simulink model "car_model"  (R2022b)
settings: Solver=VariableStepAuto  StartTime=0.0  StopTime=30  RelTol=1e-3
values from neighbouring files (symbols this model uses):
  X = Chassis_Signals.InertFrm.Cg.Disp.X.Data(:)    [Simulation_Data_Parse.m]    (also in Vehicle_Sim_Parse.m)
  Y = Chassis_Signals.InertFrm.Cg.Disp.Y.Data(:)    [Simulation_Data_Parse.m]    (also in Vehicle_Sim_Parse.m)
undefined symbols (not defined in the file or in its folder): ABS_MAX_TORQUE, ABS_MAX_TRQ_CMD, ABS_MIN_TORQUE, acc_IC, ACCELERATION_MAX, ActSuspDutyCycle, Aeq_left, Aeq_right, alpha_error, ang_acc_hystersesis, ang_IC, ang_vel_IC, area_air, axb, battery_current_IC, BATTERY_CURRENT_MAX, BATTERY_CURRENT_MIN, battery_FT_IC, battery_T_IC, BATTERY_TEMPERATURE_MAX, BATTERY_TEMPERATURE_MIN, battery_voltage_IC, BATTERY_VOLTAGE_MAX, BATTERY_VOLTAGE_MIN, Brake_Pressure_IC, ccl_IC, CENTER_STEER_ANGLE_MAX, covA, covarience_matrix_IC, covG, covM, covP, covV, cy_sweep, dB, dcl_IC, DCL_MAX, DCL_MIN, deadband_angle, dIndex, DiscIntNeverNeededParam, disk_abore, driver_t, dt_OFF, dt_ON, dTx, dx, dZ, F0z, forward_look_straight, forward_look_turn, fusion_t, fusion_t_sim, Fz_IC, Fz_sweep, g, gearbox_efficiency, gps_counter_IC, gps_ratio, gr ... (+105)
libraries: fl_lib x62, nesl_utility x16, vehdynlibtire x10, vehdynlibsuspension x8, simulink x5, autolibutils x5, sharedtransform x5, EngineCoolingComponents_lib x4, slpidlib x3, SimscapeFluids_lib x3, dspstat3 x2, shared6dof x2
(part 2 of 10)

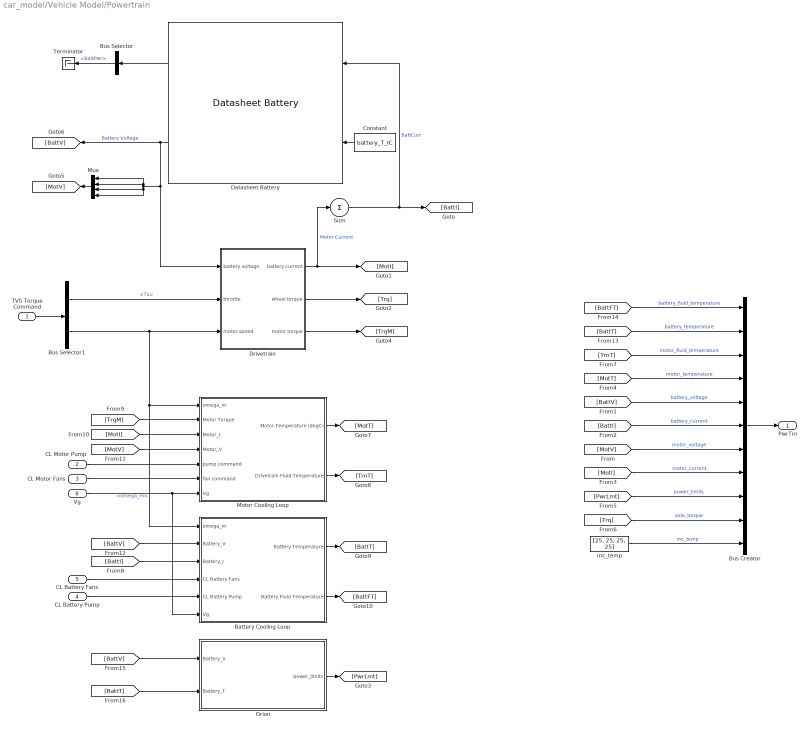
== system car_model/Vehicle Model/Powertrain ==
  TVS Torque Command : Inport
  CL Motor Pump : Inport  Port=2
  CL Motor Fans : Inport  Port=3
  CL Battery Pump : Inport  Port=4
  CL Battery Fans : Inport  Port=5
  Vg : Inport  Port=6
  Battery Cooling Loop : Subsystem
  Bus Creator : BusCreator  Inputs=11
  Bus Selector : BusSelector  OutputSignals=BattPwr
  Bus Selector1 : BusSelector  OutputSignals=Tx,omega_m
  Constant : Constant  Value=battery_T_IC
  Datasheet Battery : autolibdatasheetbattery/Datasheet Battery  CapacityCtrl=Parameter  OutputVlt=Filtered  BattChargeMax=BattCap  Em=Em  CapLUTBp=SOC  RInt=RESISTANCE  BattTempBp=TEMPERATURE  CapSOCBp=SOC  Ns=Ns  Np=Np  BattCapInit=BattCap_I  Tc=Battery_tau  Vinit=battery_voltage_IC  RefBlkName='autolibdatasheetbattery/Datasheet Battery'
  Drivetrain : Subsystem
  Motor Cooling Loop : Subsystem
  Mux : Mux
  Orion : Subsystem
  Sum : Sum  Inputs=+
  Terminator : Terminator
  mc_temp : Constant  Value=[25, 25, 25, 25]
  PwrTrn : Outport
  wires:
  [BattT] -> Orion/2(Battery_T)
  [Trq] -> Bus Creator/10  "axle_torque"
  [TrnT] -> Bus Creator/3  "motor_fluid_temperature"
  Vg/1 -> Motor Cooling Loop/7(Vg), Battery Cooling Loop/6(Vg)
  CL Battery Fans/1 -> Battery Cooling Loop/4(CL Battery Fans)
  [MotT] -> Bus Creator/4  "motor_temperature"
  Battery Cooling Loop/2(Battery Fluid Temperature) -> [BattFT]
  [BattI] -> Bus Creator/6  "battery_current"
  [MotI] -> Bus Creator/8  "motor_current"
  [MotV] -> Motor Cooling Loop/4(Motor_V)
  Motor Cooling Loop/2(Drivetrain Fluid Temperature) -> [TrnT]
  Mux/1 -> [MotV]
  CL Battery Pump/1 -> Battery Cooling Loop/5(CL Battery Pump)
  Bus Selector1/2 -> Drivetrain/3(motor speed), Motor Cooling Loop/1(omega_m), Battery Cooling Loop/1(omega_m)  "<omega_m>"
  Bus Selector1/1 -> Drivetrain/2(throttle)  "<Tx>"
  CL Motor Pump/1 -> Motor Cooling Loop/5(pump command)
  Battery Cooling Loop/1(Battery Temperature) -> [BattT]
  Sum/1 -> [BattI], Datasheet Battery/1  "BattCurr"
  Datasheet Battery/1 -> Bus Selector/1
  [BattI] -> Battery Cooling Loop/3(Battery_I)
  [BattV] -> Orion/1(Battery_V)
  Bus Selector/1 -> Terminator/1  "<BattPwr>"
  Motor Cooling Loop/1(Motor Temperature (degC)) -> [MotT]
  Datasheet Battery/2 -> Drivetrain/1(battery voltage), Mux/3, Mux/4, Mux/2, Mux/1, [BattV]  "Battery Voltage"
  [MotV] -> Bus Creator/7  "motor_voltage"
  [BattV] -> Bus Creator/5  "battery_voltage"
  [MotI] -> Motor Cooling Loop/3(Motor_I)
  [BattV] -> Battery Cooling Loop/2(Battery_V)
  [BattFT] -> Bus Creator/1  "battery_fluid_temperature"
  Drivetrain/1(battery current) -> [MotI], Sum/1  "Motor Current"
  Constant/1 -> Datasheet Battery/2
  Bus Creator/1 -> PwrTrn/1
  CL Motor Fans/1 -> Motor Cooling Loop/6(fan command)
  [PwrLmt] -> Bus Creator/9  "power_limits"
  [BattT] -> Bus Creator/2  "battery_temperature"
  Orion/1(power_limits) -> [PwrLmt]
  [TrqM] -> Motor Cooling Loop/2(Motor Torque)
  mc_temp/1 -> Bus Creator/11  "mc_temp"
  TVS Torque Command/1 -> Bus Selector1/1
  Drivetrain/2(wheel torque) -> [Trq]
  Drivetrain/3(motor torque) -> [TrqM]

== system car_model/Vehicle Model/Suspension ==
  Steering : Inport
  Wheel : Inport  Port=2
  Vehicle : Inport  Port=3
  Double Wishbone Suspension : Subsystem  VariantControl=1
      mask Display: image('suspdw.png');
  Independent Mapped Front Suspension Mapped Solid Axle Rear Suspension : Subsystem  VariantControl=2
      mask Display: image([imread('suspindmap.png');imread('suspsamap.png')]);
  Kinematics and Compliance Independent Suspension : Subsystem  VariantControl=6
      mask Display: image('suspkandc.png');
  MacPherson Front Suspension Solid Axle Rear Suspension : Subsystem  VariantControl=3
      mask Display: image([imread('suspmacp.png');imread('suspsacoil.png')]);
  MacPherson Suspension : Subsystem  VariantControl=4
      mask Display: image('suspmacp.png');
  Mapped Suspension : Subsystem  VariantControl=5
      mask Display: image('suspindmap.png');
  Suspension : Outport  VectorParamsAs1DForOutWhenUnconnected=off
  Suspension1 : Outport  Port=2  VectorParamsAs1DForOutWhenUnconnected=off
  Veh : Outport  Port=3  VectorParamsAs1DForOutWhenUnconnected=off

== system car_model/Vehicle Model/Vehicle ==
  Suspension : Inport
  6DOF : Subsystem  VariantControl=1
  Constant : Constant  Value=[0 0 0]
  VehFdbk : Outport  VectorParamsAs1DForOutWhenUnconnected=off
  wires:
  6DOF/1(VehFdbk) -> VehFdbk/1  "VehFdbk"
  Constant/1 -> 6DOF/2(Wind)
  Suspension/1 -> 6DOF/1(Suspension)

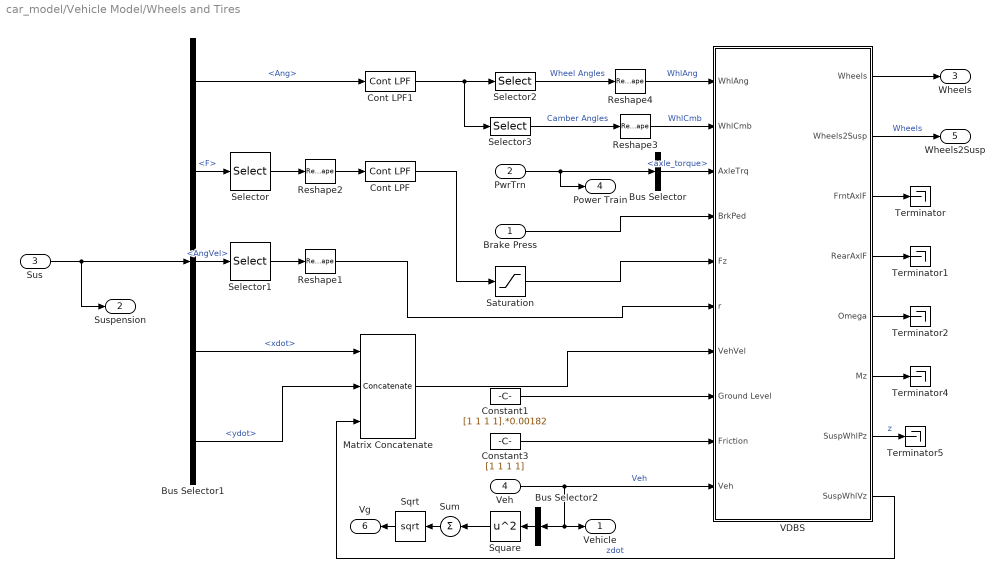
== system car_model/Vehicle Model/Wheels and Tires ==
  Brake Press : Inport  Unit=Pa
  PwrTrn : Inport  Port=2
  Sus : Inport  Port=3
  Veh : Inport  Port=4
  Bus Selector : BusSelector  OutputSignals=axle_torque
  Bus Selector1 : BusSelector  OutputSignals=Whl.Ang,Whl.F,Whl.AngVel,Whl.xdot,Whl.ydot
  Bus Selector2 : BusSelector  OutputSignals=BdyFrm.Cg.Vel.xdot,BdyFrm.Cg.Vel.ydot  OutputAsBus=on
  Constant1 : Constant  Value=[1 1 1 1].*0.00182
  Constant3 : Constant  Value=[1 1 1 1]
  Cont LPF : autolibutils/Cont LPF  wc=100*2*pi  AbsoluteTolerance=auto  aMode=2
  Cont LPF1 : autolibutils/Cont LPF  wc=100*2*pi  AbsoluteTolerance=auto  aMode=2
  Matrix Concatenate : Concatenate  NumInputs=3  Mode=Multidimensional array
  Reshape{1..4} (4 alike) : Reshape
  Saturation : Saturate  UpperLimit=inf  LowerLimit=-10*9.81*2000  ZeroCross=off
  Selector : Selector  NumberOfDimensions=2  InputPortWidth=3  IndexOptions=Index vector (dialog),Select all  Indices=[3],1  OutputSizes=1,1
  Selector1 : Selector  NumberOfDimensions=2  InputPortWidth=1  IndexOptions=Index vector (dialog),Select all  Indices=[3],1  OutputSizes=1,1
  Selector2 : Selector  NumberOfDimensions=2  InputPortWidth=3  IndexOptions=Index vector (dialog),Select all  Indices=3,1  OutputSizes=1,1
  Selector3 : Selector  NumberOfDimensions=2  InputPortWidth=3  IndexOptions=Index vector (dialog),Select all  Indices=1,1  OutputSizes=1,1
  Sqrt : Sqrt
  Square : Math  Operator=square
  Sum : Sum  Inputs=+
  Terminator{,1..2,4..5} (5 alike) : Terminator
  VDBS : Subsystem  VariantControl=0
  Vehicle : Outport  VectorParamsAs1DForOutWhenUnconnected=off
  Suspension : Outport  Port=2  VectorParamsAs1DForOutWhenUnconnected=off
  Wheels : Outport  Port=3  VectorParamsAs1DForOutWhenUnconnected=off
  Power Train : Outport  Port=4  VectorParamsAs1DForOutWhenUnconnected=off
  Wheels2Susp : Outport  Port=5  VectorParamsAs1DForOutWhenUnconnected=off
  Vg : Outport  Port=6  VectorParamsAs1DForOutWhenUnconnected=off
  wires:
  Bus Selector1/2 -> Selector/1  "<F>"
  VDBS/3(FrntAxlF) -> Terminator/1
  VDBS/4(RearAxlF) -> Terminator1/1
  VDBS/6(Mz) -> Terminator4/1
  Selector1/1 -> Reshape1/1
  Matrix Concatenate/1 -> VDBS/7(VehVel)
  PwrTrn/1 -> Power Train/1, Bus Selector/1
  Reshape4/1 -> VDBS/1(WhlAng)  "WhlAng"
  Reshape3/1 -> VDBS/2(WhlCmb)  "WhlCmb"
  Selector/1 -> Reshape2/1
  Saturation/1 -> VDBS/5(Fz)
  Constant1/1 -> VDBS/8(Ground Level)
  VDBS/8(SuspWhlVz) -> Matrix Concatenate/3  "zdot"
  Bus Selector1/1 -> Cont LPF1/1  "<Ang>"
  Selector3/1 -> Reshape3/1  "Camber Angles"
  Sus/1 -> Suspension/1, Bus Selector1/1
  Bus Selector1/4 -> Matrix Concatenate/1  "<xdot>"
  Bus Selector1/5 -> Matrix Concatenate/2  "<ydot>"
  VDBS/7(SuspWhlPz) -> Terminator5/1  "z"
  Reshape2/1 -> Cont LPF/1
  Bus Selector1/3 -> Selector1/1  "<AngVel>"
  Reshape1/1 -> VDBS/6(r)
  Brake Press/1 -> VDBS/4(BrkPed)
  Constant3/1 -> VDBS/9(Friction)
  Cont LPF/1 -> Saturation/1
  Cont LPF1/1 -> Selector3/1, Selector2/1
  Selector2/1 -> Reshape4/1  "Wheel Angles"
  Veh/1 -> Vehicle/1, Bus Selector2/1, VDBS/10(Veh)  "Veh"
  VDBS/2(Wheels2Susp) -> Wheels2Susp/1  "Wheels"
  VDBS/1(Wheels) -> Wheels/1
  Bus Selector/1 -> VDBS/3(AxleTrq)  "<axle_torque>"
  VDBS/5(Omega) -> Terminator2/1
  Bus Selector2/1 -> Square/1
  Square/1 -> Sum/1
  Sum/1 -> Sqrt/1
  Sqrt/1 -> Vg/1

== system car_model/Control Systems/TVS/Current Limiting ==
  max_K : Inport
  omega : Inport  Port=2
  Tx : Inport  Port=3
  Divide : Product  Inputs=/**
  Gain : Gain  Gain=1./ABS_MAX_TORQUE
  Gain1 : Gain  Gain=PER23_gr
  Gain2 : Gain  Gain=MOTOR_ENABLE
  GreaterThan : RelationalOperator  Operator=<  OutDataTypeStr=boolean  RndMeth=Simplest  InputSameDT=off
  Max : MinMax  Function=max
  Max K : Lookup_n-D  NumberOfTableDimensions=1  BreakpointsForDimension1=[0 675]  Table=[0.05 1]  ExtrapMethod=Clip  UseLastTableValue=on  InternalRulePriority=Speed  RndMeth=Simplest
  Min K : Lookup_n-D  NumberOfTableDimensions=1  BreakpointsForDimension1=[0 100 200 1150]  IndexSearchMethod=Linear search  Table=[0 0 0.1 1]  ExtrapMethod=Clip  UseLastTableValue=on  InternalRulePriority=Speed  RndMeth=Simplest
  Product : Product
  Sum : Sum  Inputs=+
  Sum1 : Sum  Inputs=+|+
  Sum2 : Sum  Inputs=|+-
  Switch : Switch  Criteria=u2 > Threshold  SaturateOnIntegerOverflow=off  InputSameDT=off
  K_Actual : Outport
  wires:
  max_K/1 -> Divide/3, GreaterThan/1
  Switch/1 -> K_Actual/1
  Gain/1 -> Product/1
  Tx/1 -> Gain/1
  GreaterThan/1 -> Sum/1
  Sum/1 -> Switch/2
  omega/1 -> Gain1/1
  Min K/1 -> Gain2/1, Sum2/2
  Max K/1 -> Sum2/1
  Sum2/1 -> Product/2
  Product/1 -> Sum1/1
  Sum1/1 -> Switch/3, Divide/2, Max/1, GreaterThan/2
  Max/1 -> Divide/1
  Divide/1 -> Switch/1
  Gain1/1 -> Min K/1, Max K/1
  Gain2/1 -> Sum1/2

== system car_model/Control Systems/TVS/Optimization ==
  note: reduce this limit?
  driver_input : Inport  OutDataTypeStr=double
  obj_gain : Inport  Port=2
  b : Inport  Port=3  OutDataTypeStr=double
  ub : Inport  Port=4  OutDataTypeStr=double
  lb : Inport  Port=5  OutDataTypeStr=double
  Aeq : Inport  Port=6  OutDataTypeStr=double
  beq : Inport  Port=7  OutDataTypeStr=double
  A Dot : DotProduct  OutDataTypeStr=double
  Aeq Dot : DotProduct  OutDataTypeStr=double
  C Caller : CCaller  FunctionName=bigM_func  PortSpecificationStruct="%)30     .    N\"X   8    (     @         %    \"    !P    !     0         %  0 \"0    $    _    07)G3F%M90  4&]R=$YA;64 4V-O<&4     26YD97@     5'EP90      4VEZ90      27-';&]B86P   X    P    !@    @    $          4    (     0    ,    !         !   P!O=70 #@   #     &    \"     0         !0    @    !     P    $         $  # &]U=  .    .     8    (    !          %    \"     $    &     0         0  ...(+15750 chars)"
  Constant : Constant  Value=TVS_ENABLE
  Constant1 : Constant  Value=[1 1 1 1]
  Demux{,1..4} (5 alike) : Demux
  Switch : Switch  Criteria=u2 > Threshold  SaturateOnIntegerOverflow=off  InputSameDT=off
  Tx_RAW_demux : Mux
  Tx_choose : Switch  Criteria=u2 > Threshold  Threshold=2  OutDataTypeStr=double  SaturateOnIntegerOverflow=off  InputSameDT=off
  Tx_deadband : DeadZone  LowerValue=-10*dTx  UpperValue=10*dTx  SaturateOnIntegerOverflow=off
  Tx_equal_gain : Gain  Gain=ABS_MAX_TORQUE.*MOTOR_ENABLE  OutDataTypeStr=double
  Tx_equal_offset : Bias  Bias=ABS_MAX_TORQUE  SaturateOnIntegerOverflow=off
  Tx_initial : Constant  Value=Tx_I  OutDataTypeStr=double
  Tx_reverse_offset : Bias  Bias=-ABS_MAX_TORQUE  SaturateOnIntegerOverflow=off
  b Add : Sum  OutDataTypeStr=double
  beq Add : Sum  OutDataTypeStr=double
  lb_offset : Bias  Bias=ABS_MAX_TORQUE  SaturateOnIntegerOverflow=off
  optimization_offset_A : Constant  Value=ABS_MAX_TORQUE  OutDataTypeStr=double
  optimization_offset_Aeq : Constant  Value=ABS_MAX_TORQUE  OutDataTypeStr=double
  ub_offset : Bias  Bias=ABS_MAX_TORQUE  SaturateOnIntegerOverflow=off
  yaw_error_limit : Constant  Value=yaw_error_limit  OutDataTypeStr=double
  Tx : Outport
  exitflag : Outport  Port=2
  wires:
  C Caller/1 -> Tx_choose/2, exitflag/1  "exitflag"
  lb/1 -> lb_offset/1  "lb"
  ub/1 -> ub_offset/1  "ub"
  C Caller/2 -> Tx_RAW_demux/1  "TFL"
  C Caller/5 -> Tx_RAW_demux/4  "TRR"
  C Caller/4 -> Tx_RAW_demux/3  "TRL"
  C Caller/3 -> Tx_RAW_demux/2  "TFR"
  Demux/1 -> C Caller/1  "obj_FL"
  Demux/2 -> C Caller/2  "obj_FR"
  Demux/3 -> C Caller/3  "obj_RL"
  Demux/4 -> C Caller/4  "obj_RR"
  Tx_initial/1 -> C Caller/23, C Caller/24, C Caller/25, C Caller/26  "Tx_initial"
  Demux1/1 -> C Caller/19  "ub_FL"
  Demux1/2 -> C Caller/20  "ub_FR"
  Demux1/3 -> C Caller/21  "ub_RL"
  Demux1/4 -> C Caller/22  "ub_RR"
  Demux2/1 -> C Caller/15  "lb_FL"
  Demux2/2 -> C Caller/16  "lb_FR"
  Demux2/3 -> C Caller/17  "lb_RL"
  Demux2/4 -> C Caller/18  "lb_RR"
  Demux3/3 -> C Caller/13  "Aeq_RL"
  Demux3/2 -> C Caller/12  "Aeq_FR"
  Demux3/1 -> C Caller/11  "Aeq_FL"
  Demux3/4 -> C Caller/14  "Aeq_RR"
  Demux4/1 -> C Caller/6  "A_FL"
  Demux4/2 -> C Caller/7  "A_FR"
  Demux4/3 -> C Caller/8  "A_RL"
  Demux4/4 -> C Caller/9  "A_RR"
  ub_offset/1 -> Demux1/1  "ub_b"
  optimization_offset_Aeq/1 -> Aeq Dot/1  "offset"
  optimization_offset_A/1 -> A Dot/1  "offset"
  beq/1 -> beq Add/1  "beq"
  Aeq Dot/1 -> beq Add/2  "Aeq_b"
  b/1 -> b Add/1  "b"
  A Dot/1 -> b Add/2
  yaw_error_limit/1 -> C Caller/27  "yaw_error_limit"
  Tx_RAW_demux/1 -> Tx_choose/1  "Tx_RAW_TV"
  Constant1/1 -> Demux4/1, A Dot/2  "A"
  b Add/1 -> C Caller/5  "b_b"
  obj_gain/1 -> Demux/1  "obj_gain"
  lb_offset/1 -> Demux2/1  "lb_b"
  Aeq/1 -> Demux3/1, Aeq Dot/2  "Aeq"
  beq Add/1 -> C Caller/10  "beq_b"
  Tx_deadband/1 -> Tx/1  "Tx"
  Tx_reverse_offset/1 -> Tx_deadband/1
  driver_input/1 -> Tx_equal_gain/1
  Tx_choose/1 -> Switch/1
  Tx_equal_gain/1 -> Tx_equal_offset/1  "Tx_equal"
  Tx_equal_offset/1 -> Switch/3, Tx_choose/3
  Switch/1 -> Tx_reverse_offset/1
  Constant/1 -> Switch/2

== system car_model/Control Systems/TVS/Power Controller ==
  note: Max Throttle as Limit or Max Current as limit?
  note: Tune the endpoints
  vel : Inport  OutDataTypeStr=double
  battery_voltage : Inport  Port=2
  dcl : Inport  Port=3  OutDataTypeStr=double  LockScale=on
  ccl : Inport  Port=4  OutDataTypeStr=double  LockScale=on
  driver_input : Inport  Port=5  OutDataTypeStr=double  LockScale=on
  motor_temp : Inport  Port=6
  mc_temp : Inport  Port=7
  omega : Inport  Port=8
  In9 : Inport  Port=9
  Constant2 : Constant  Value=[0 0 0 0]  OutDataTypeStr=double
  Constant3 : Constant  Value=ABS_MAX_TORQUE
  Current to RAW Throttle : Gain  Gain=1/(2*MOTOR_CURRENT_LIMIT)
  Gain : Gain  Gain=2*MOTOR_CURRENT_LIMIT
  Gain1 : Gain  Gain=ABS_MAX_TRQ_CMD
  Gain4 : Gain  Gain=-MOTOR_ENABLE  ParamDataTypeStr=double  OutDataTypeStr=Inherit: Inherit via back propagation
  Gain8 : Gain  Gain=MOTOR_ENABLE  ParamDataTypeStr=double  OutDataTypeStr=Inherit: Inherit via back propagation
  Max : MinMax  Function=max
  Max Torque : Saturate  UpperLimit=ABS_MAX_TORQUE  LowerLimit=dTx  OutDataTypeStr=Inherit: Inherit via back propagation
  Max1 : MinMax  Function=max
  Min Torque : Saturate  UpperLimit=ABS_MIN_TORQUE  LowerLimit=0  OutDataTypeStr=Inherit: Inherit via back propagation
  Minimum : MinMax  Inputs=4
  Saturation : Saturate  UpperLimit=ABS_MAX_TRQ_CMD  LowerLimit=dTx*10
  Selector : Selector  InputPortWidth=4  IndexOptions=Index vector (dialog)  Indices=4  OutputSizes=1
  Switch1 : Switch  Threshold=min_velocity_regen  OutDataTypeStr=Inherit: Inherit via back propagation  SaturateOnIntegerOverflow=off  InputSameDT=off
  Temperature to Motor Controller Current Limit Map : Lookup_n-D  NumberOfTableDimensions=1  BreakpointsForDimension1=motorControllerCurve(:,1)  IndexSearchMethod=Evenly spaced points  Table=motorControllerCurve(:,2)  ExtrapMethod=Clip  UseLastTableValue=on  InternalRulePriority=Speed  RndMeth=Simplest
  Temperature to Motor Current Limit Map : Lookup_n-D  NumberOfTableDimensions=1  BreakpointsForDimension1=motorTempX  IndexSearchMethod=Evenly spaced points  Table=motorTempCurve  ExtrapMethod=Clip  UseLastTableValue=on  InternalRulePriority=Speed  RndMeth=Simplest
  Terminator : Terminator
  Terminator1 : Terminator
  Terminator2 : Terminator
  b : Outport  OutDataTypeStr=double  LockScale=on
  max_K : Outport  Port=2  OutDataTypeStr=double  LockScale=on
  ub : Outport  Port=3  OutDataTypeStr=double  LockScale=on
  lb : Outport  Port=4  OutDataTypeStr=double  LockScale=on
  wires:
  Max1/1 -> Temperature to Motor Controller Current Limit Map/1
  Temperature to Motor Current Limit Map/1 -> Minimum/2  "Total Motor Current Limit (A)"
  battery_voltage/1 -> Terminator1/1
  Gain8/1 -> Max Torque/1
  Constant3/1 -> Gain4/1, Gain8/1
  Saturation/1 -> b/1  "Limited Total Torque Request (Nm)"
  Max/1 -> Temperature to Motor Current Limit Map/1
  Gain4/1 -> Min Torque/1
  Constant2/1 -> Switch1/3  "Abs Min Torque CMD"
  Selector/1 -> Switch1/2  "Planer Vcog (m/s)"
  motor_temp/1 -> Max/1  "[FL FR RL RR] Motor Temperature (degC)"
  ccl/1 -> Terminator/1
  driver_input/1 -> Gain/1, Gain1/1  "RAW Throttle"
  Max Torque/1 -> ub/1  "Max Individual Motor Torque (Nm)"
  Gain/1 -> Minimum/1
  mc_temp/1 -> Max1/1  "[FL FR RL RR] Motor Controller Temperature (degC)"
  dcl/1 -> Minimum/4  "Discharge Current Limit (A)"
  vel/1 -> Selector/1  "[Vx Vy Vcog]"
  Temperature to Motor Controller Current Limit Map/1 -> Minimum/3  "Total Motor Controller Current Limit (A)"
  Min Torque/1 -> Switch1/1
  Switch1/1 -> lb/1  "Min Individual Motor Torque (Nm)"
  Minimum/1 -> Current to RAW Throttle/1  "Max Allowed Current (A)"
  omega/1 -> Terminator2/1
  Gain1/1 -> Saturation/1
  Current to RAW Throttle/1 -> max_K/1  "Torque CMD (none)"

== system car_model/Control Systems/TVS/Traction Controller ==
  Fz : Inport  OutDataTypeStr=double  LockScale=on
  vel : Inport  Port=2  OutDataTypeStr=double  LockScale=on
  ang_vel : Inport  Port=3  OutDataTypeStr=double  LockScale=on
  CCSA : Inport  Port=4
  omega : Inport  Port=5
  1-D Lookup Table : Lookup_n-D  NumberOfTableDimensions=1  BreakpointsForDimension1=Fz_sweep  Table=cy_sweep  InternalRulePriority=Speed  RndMeth=Simplest
  1-D Lookup Table1 : Lookup_n-D  NumberOfTableDimensions=1  BreakpointsForDimension1=Fz_sweep  Table=my_sweep  InternalRulePriority=Speed  RndMeth=Simplest
  1-D Lookup Table2 : Lookup_n-D  NumberOfTableDimensions=1  BreakpointsForDimension1=Fz_sweep  Table=kx_sweep  InternalRulePriority=Speed  RndMeth=Simplest
  1-D Lookup Table3 : Lookup_n-D  NumberOfTableDimensions=1  BreakpointsForDimension1=Fz_sweep  Table=mx_sweep  InternalRulePriority=Speed  RndMeth=Simplest
  Compute SA : Subsystem
  Compute SL : Subsystem
  Compute SL Fake : Subsystem
  Constant : Constant
  Constant1 : Constant  Value=[1 1 1 1].*low_V_SA
  Constant2 : Constant  Value=TRACTION_ENABLE
  Divide : Product  Inputs=**//
  Divide1 : Product  Inputs=**//
  Gain : Gain  Gain=gr./RE
  Selector : Selector  InputPortWidth=4  IndexOptions=Index vector (dialog)  Indices=4  OutputSizes=1
  Selector1 : Selector  InputPortWidth=4  IndexOptions=Index vector (dialog)  Indices=4  OutputSizes=1
  Sqrt : Sqrt
  Square : Math  Operator=square
  Square1 : Math  Operator=square
  Steering Model : Subsystem
  Sum : Sum  Inputs=|++
  Switch : Switch  Criteria=u2 > Threshold  Threshold=Vth  SaturateOnIntegerOverflow=off  InputSameDT=off
  Switch1 : Switch  Criteria=u2 > Threshold  Threshold=Vth  SaturateOnIntegerOverflow=off  InputSameDT=off
  Switch2 : Switch  Criteria=u2 > Threshold  SaturateOnIntegerOverflow=off  InputSameDT=off
  obj_gain : Outport
  wires:
  Gain/1 -> obj_gain/1  "obj_gain"
  Constant/1 -> Gain/1, Switch2/3
  Sum/1 -> Sqrt/1
  Divide/1 -> Square/1  "a_bar"
  1-D Lookup Table/1 -> Divide/2
  1-D Lookup Table1/1 -> Divide/3
  Fz/1 -> 1-D Lookup Table1/1, Divide/4, 1-D Lookup Table2/1, 1-D Lookup Table3/1, Divide1/4, 1-D Lookup Table/1
  Divide1/1 -> Square1/1  "s_bar"
  1-D Lookup Table2/1 -> Divide1/2
  1-D Lookup Table3/1 -> Divide1/3
  Switch/1 -> Divide1/1
  Switch1/1 -> Divide/1
  Compute SL Fake/1(SL_fake) -> Switch/3
  Compute SL/1(Out1) -> Switch/1
  Compute SA/1(Out1) -> Switch1/1, Compute SL/1(In1)
  vel/1 -> Compute SL/3(Vg), Selector/1, Compute SL Fake/2(Vg), Selector1/1, Compute SA/3(Vg)
  ang_vel/1 -> Compute SA/2(ang_vel)
  omega/1 -> Compute SL Fake/1(omega), Compute SL/2(omega)
  Steering Model/1(steering) -> Compute SA/1(steering)
  Constant1/1 -> Switch1/3
  Sqrt/1 -> Switch2/1
  Constant2/1 -> Switch2/2
  Selector/1 -> Switch/2
  Selector1/1 -> Switch1/2
  Square/1 -> Sum/1
  Square1/1 -> Sum/2
  CCSA/1 -> Steering Model/1(steering_angle)

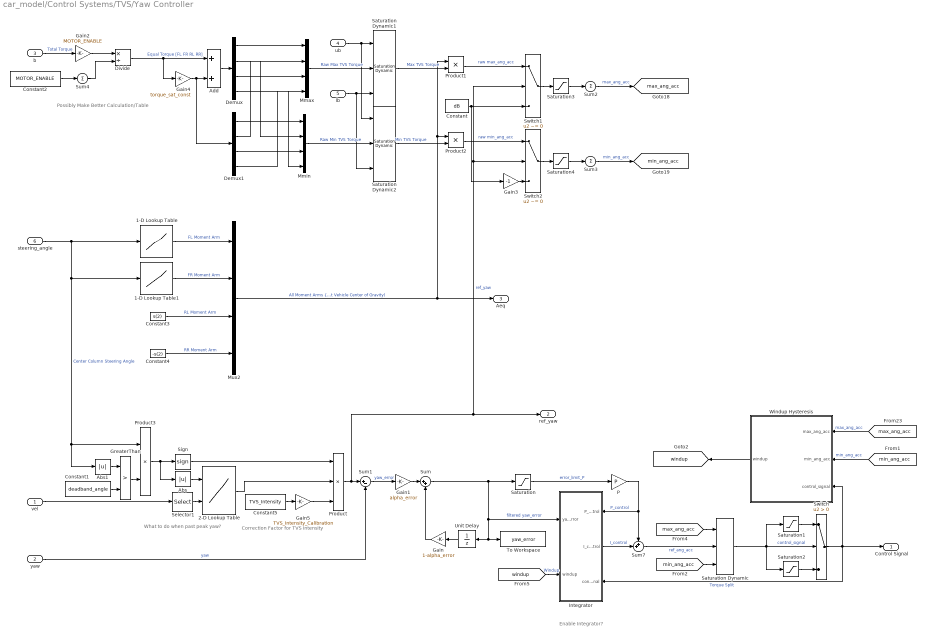
== system car_model/Control Systems/TVS/Yaw Controller ==
  note: Correction Factor for TVS Intensity
  note: Enable Integrator?
  note: What to do when past peak yaw?
  note: Possibly Make Better Calculation/Table
  vel : Inport
  yaw : Inport  Port=2  OutDataTypeStr=double  LockScale=on
  b : Inport  Port=3
  ub : Inport  Port=4
  lb : Inport  Port=5
  steering_angle : Inport  Port=6
  1-D Lookup Table : Lookup_n-D  NumberOfTableDimensions=1  BreakpointsForDimension1=theta_sweep  Table=Aeq_left  ExtrapMethod=Clip  InternalRulePriority=Speed  RndMeth=Simplest
  1-D Lookup Table1 : Lookup_n-D  NumberOfTableDimensions=1  BreakpointsForDimension1=theta_sweep  Table=Aeq_right  ExtrapMethod=Clip  InternalRulePriority=Speed  RndMeth=Simplest
  2-D Lookup Table : Lookup_n-D  BreakpointsForDimension1=steering_sweep  BreakpointsForDimension2=velocity_sweep  Table=yaw_rate  ExtrapMethod=Clip  InternalRulePriority=Speed  RndMeth=Simplest
      settings: InputPortMap=u0,u1
  Abs : Abs  SaturateOnIntegerOverflow=off
  Abs1 : Abs  SaturateOnIntegerOverflow=off
  Add : Sum
  Constant : Constant  Value=dB  OutDataTypeStr=Inherit: Inherit via back propagation
  Constant1 : Constant  Value=deadband_angle
  Constant2 : Constant  Value=MOTOR_ENABLE
  Constant3 : Constant  Value=s(2)  OutDataTypeStr=Inherit: Inherit via back propagation
  Constant4 : Constant  Value=-s(2)  OutDataTypeStr=Inherit: Inherit via back propagation
  Constant5 : Constant  Value=TVS_Intensity
  Demux : Demux
  Demux1 : Demux
  Divide : Product  Inputs=*/
  Gain : Gain  Gain=1-alpha_error
  Gain1 : Gain  Gain=alpha_error
  Gain2 : Gain  Gain=MOTOR_ENABLE
  Gain3 : Gain  Gain=-1
  Gain4 : Gain  Gain=torque_sat_const
  Gain5 : Gain  Gain=TVS_Intensity_Calibration
  GreaterThan : RelationalOperator  Operator=>  OutDataTypeStr=boolean  RndMeth=Simplest  InputSameDT=off
  Integrator : Subsystem
      settings: PortSchema="{\"entries\":[{\"content\":{\"sides\":[{\"content\":{\"connectorIds\":[\"In1\",\"In2\"]},\"type\":\"ConnectorPlacement.EquallySpacedRectSide\",\"uuid\":\"8eceed30-5463-482b-9ad9-1d0859eec1e0\"},{\"content\":{\"connectorIds\":[\"In3\",\"Out1\",\"In4\"],\"side\":\"RIGHT\"},\"type\":\"ConnectorPlacement.EquallySpacedRectSide\",\"uuid\":\"ca18b8b2-b2b4-4da4-8362-ca68ae703b33\"},{\"content\":{\"connectorIds\":[],\"side\":\"TOP\"},\"type\":\"ConnectorPlacement.EquallySpacedRectSide\",\"uuid\":\"14e81d29-e47e-408e-961b-b14eadc3d40e\"}]},\"type\":\"ConnectorPlacement.EquallySpacedConnector\",\"uuid\":\"147d3fcd-d0df-4d8b-910b-d1c7e2c77e1f\"}],\"packageUris\":[\"http://schema.mathworks.com/mf0/Connector/R2020b\"],\"version\":\"1.0\"}"
  Mmax : Mux
  Mmin : Mux
  Mux2 : Mux
  P : Gain  Gain=P  ParamDataTypeStr=double  OutDataTypeStr=double
  Product : Product  Inputs=3  OutDataTypeStr=Inherit: Inherit via back propagation
  Product1 : Product
  Product2 : Product
  Product3 : Product
  Saturation : Saturate  UpperLimit=YAW_MAX  LowerLimit=-YAW_MAX
  Saturation Dynamic : simulink/Discontinuities/Saturation Dynamic  OutMin=[]  OutMax=[]  OutDataTypeStr=Inherit: Same as second input  OutDataType=fixdt(1, 16)  OutScaling=2^-10  DoSatur=off
  Saturation Dynamic1 : simulink/Discontinuities/Saturation Dynamic  OutMin=[]  OutMax=[]  OutDataTypeStr=Inherit: Same as second input  OutDataType=fixdt(1, 16)  OutScaling=2^-10  DoSatur=off
  Saturation Dynamic2 : simulink/Discontinuities/Saturation Dynamic  OutMin=[]  OutMax=[]  OutDataTypeStr=Inherit: Same as second input  OutDataType=fixdt(1, 16)  OutScaling=2^-10  DoSatur=off
  Saturation1 : Saturate  UpperLimit=inf  LowerLimit=dB
  Saturation2 : Saturate  UpperLimit=-dB  LowerLimit=-inf
  Saturation3 : Saturate  UpperLimit=inf  LowerLimit=dB
  Saturation4 : Saturate  UpperLimit=-dB  LowerLimit=-inf
  Selector1 : Selector  InputPortWidth=4  IndexOptions=Index vector (dialog)  Indices=4  OutputSizes=1
  Sign : Signum
  Sum : Sum  Inputs=|++
  Sum1 : Sum  Inputs=|+-  OutDataTypeStr=Inherit: Inherit via back propagation
  Sum2 : Sum  Inputs=+
  Sum3 : Sum  Inputs=+
  Sum4 : Sum  Inputs=+
  Sum7 : Sum  Inputs=++|  OutDataTypeStr=double  SaturateOnIntegerOverflow=on
  Switch : Switch  Criteria=u2 > Threshold  SaturateOnIntegerOverflow=off  InputSameDT=off
  Switch1 : Switch  Criteria=u2 ~= 0  OutDataTypeStr=Inherit: Inherit via back propagation  SaturateOnIntegerOverflow=off  InputSameDT=off
  Switch2 : Switch  Criteria=u2 ~= 0  OutDataTypeStr=Inherit: Inherit via back propagation  SaturateOnIntegerOverflow=off  InputSameDT=off
  To Workspace : ToWorkspace  VariableName=yaw_error  SaveFormat=Timeseries  SampleTime=-1
  Unit Delay : UnitDelay  SampleTime=-1  HasFrameUpgradeWarning=on
  Windup Hysteresis : Subsystem
  Control Signal : Outport  OutDataTypeStr=double  PortDimensions=1  LockScale=on
  ref_yaw : Outport  Port=2
  Aeq : Outport  Port=3  OutDataTypeStr=double  LockScale=on
  tag scope: max_ang_acc=global, min_ang_acc=global, windup=global
  wires:
  P/1 -> Sum7/1, Integrator/3(P_control)  "P_control"
  yaw/1 -> Sum1/2  "yaw"
  Integrator/1(I_control) -> Sum7/2  "I_control"
  Sum7/1 -> Saturation Dynamic/2  "ref_ang_acc"
  Saturation Dynamic/1 -> Saturation2/1, Saturation1/1, Switch/2  "control_signal"
  Sum2/1 -> [max_ang_acc]  "max_ang_acc"
  Sum3/1 -> [min_ang_acc]  "min_ang_acc"
  Saturation/1 -> P/1  "error_limit_P"
  Windup Hysteresis/1(windup) -> [windup]
  Sum/1 -> Saturation/1, Unit Delay/1, To Workspace/1, Integrator/1(yaw_error)  "filtered yaw_error"
  [windup] -> Integrator/2(windup)  "Windup"
  Unit Delay/1 -> Gain/1
  Gain/1 -> Sum/2
  Gain1/1 -> Sum/1
  Sum1/1 -> Gain1/1  "yaw_error"
  Switch/1 -> Windup Hysteresis/3(control_signal), Control Signal/1, Integrator/4(control_signal)  "Torque Split"
  Saturation1/1 -> Switch/1
  Saturation2/1 -> Switch/3
  Saturation4/1 -> Sum3/1
  Gain3/1 -> Switch2/3
  Demux1/4 -> Mmax/4
  Constant4/1 -> Mux2/4  "RR Moment Arm"
  Switch2/1 -> Saturation4/1
  b/1 -> Gain2/1  "Total Torque"
  Constant3/1 -> Mux2/3  "RL Moment Arm"
  1-D Lookup Table/1 -> Mux2/1  "FL Moment Arm"
  Demux/3 -> Mmax/3
  Gain4/1 -> Demux1/1, Add/2
  Demux1/3 -> Mmin/3
  Product1/1 -> Switch1/1  "raw max_ang_acc"
  Demux/4 -> Mmin/4
  1-D Lookup Table1/1 -> Mux2/2  "FR Moment Arm"
  Demux/2 -> Mmin/2
  Mux2/1 -> Aeq/1, Product2/1, Product1/1  "All Moment Arms {FL FR RL RR] (about Vehicle Center of Gravity)"
  Demux/1 -> Mmax/1
  Add/1 -> Demux/1
  Demux1/2 -> Mmax/2
  ub/1 -> Saturation Dynamic2/1, Saturation Dynamic1/1
  Saturation Dynamic1/1 -> Product1/2  "Max TVS Torque"
  Demux1/1 -> Mmin/1
  lb/1 -> Saturation Dynamic2/3, Saturation Dynamic1/3
  Product2/1 -> Switch2/1  "raw min_ang_acc"
  Mmax/1 -> Saturation Dynamic1/2  "Raw Max TVS Torque"
  Constant/1 -> Switch1/3, Gain3/1
  Saturation3/1 -> Sum2/1
  Mmin/1 -> Saturation Dynamic2/2  "Raw Min TVS Torque"
  Saturation Dynamic2/1 -> Product2/2  "Min TVS Torque"
  Divide/1 -> Gain4/1, Add/1  "Equal Torque [FL FR RL RR]"
  Switch1/1 -> Saturation3/1
  Product/1 -> ref_yaw/1, Switch2/2, Switch1/2, Sum1/1  "ref_yaw"
  Constant1/1 -> GreaterThan/2
  steering_angle/1 -> 1-D Lookup Table1/1, Abs1/1, Product3/1, 1-D Lookup Table/1  "Center Column Steering Angle"
  vel/1 -> Selector1/1
  Abs/1 -> 2-D Lookup Table/1
  Product3/1 -> Abs/1, Sign/1
  Sign/1 -> Product/1
  Abs1/1 -> GreaterThan/1
  GreaterThan/1 -> Product3/2
  Selector1/1 -> 2-D Lookup Table/2
  [min_ang_acc] -> Windup Hysteresis/2(min_ang_acc)  "min_ang_acc"
  [max_ang_acc] -> Windup Hysteresis/1(max_ang_acc)  "max_ang_acc"
  [min_ang_acc] -> Saturation Dynamic/3
  [max_ang_acc] -> Saturation Dynamic/1
  Constant5/1 -> Gain5/1
  2-D Lookup Table/1 -> Product/2
  Gain5/1 -> Product/3
  Constant2/1 -> Sum4/1
  Gain2/1 -> Divide/1
  Sum4/1 -> Divide/2

== system car_model/Driver & Environment/Longitudinal Control/AAS ==
  v_error : Inport
  Abs : Abs  SaturateOnIntegerOverflow=off
  Constant : Constant
  Discrete-Time Integrator : DiscreteIntegrator  ExternalReset=rising  SampleTime=-1  LimitOutput=on  UpperSaturationLimit=MAX_I_Driver  LowerSaturationLimit=-MAX_I_Driver  ICPrevOutput=DiscIntNeverNeededParam  ICPrevScaledInput=DiscIntNeverNeededParam
  Gain : Gain  Gain=P_Driver
  Gain1 : Gain  Gain=I_Driver
  Less Than : RelationalOperator  Operator=<  OutDataTypeStr=boolean  RndMeth=Simplest  InputSameDT=off
  NOT : Logic  Operator=NOT  IconShape=distinctive  AllPortsSameDT=off  OutDataTypeStr=boolean
  Product : Product
  Saturation : Saturate  UpperLimit=Max_Driver_Input  LowerLimit=Min_Driver_Input
  Sum2 : Sum  Inputs=|++
  driver_input : Outport
  wires:
  Constant/1 -> Less Than/2
  Gain1/1 -> Discrete-Time Integrator/1
  Gain/1 -> Saturation/1, Sum2/1
  Discrete-Time Integrator/1 -> Sum2/2
  Less Than/1 -> NOT/1, Product/2
  NOT/1 -> Discrete-Time Integrator/2
  Abs/1 -> Less Than/1
  Product/1 -> Gain1/1
  Saturation/1 -> driver_input/1
  v_error/1 -> Abs/1, Product/1, Gain/1  "v_error"

== system car_model/Driver & Environment/Longitudinal Control/ABS ==
  omega : Inport
  In2 : Inport  Port=2
  <v_error> : Inport  Port=3
  In3 : Inport  Port=4
  ABS_ENABLE : Inport  Port=5
  2-D Lookup Table : Lookup_n-D  BreakpointsForDimension1=[0;20;80;130]  BreakpointsForDimension2=[200;400;1000;1200]  Table=[0 500000 2000000 3000000;0 250000 1500000 2000000;0 200000 1000000 1500000;0 100000 500000 1000000]  InternalRulePriority=Speed  RndMeth=Simplest
      settings: InputPortMap=u0,u1
  Abs : Abs  SaturateOnIntegerOverflow=off
  Bias : Bias  Bias=2000000  SaturateOnIntegerOverflow=off
  Dead Zone : DeadZone  LowerValue=-20  UpperValue=20
  Discrete Derivative : simulink/Discrete/Discrete Derivative  gainval=1.0  ICPrevScaledInput=0.0  OutMin=[]  OutMax=[]  OutDataType=fixdt(1, 16)  OutScaling=2^-10  DoSatur=off
  Gain : Gain  Gain=4/(mu_kinetic*pi*Rm*num_pads*disk_abore^2)
  Gain1 : Gain  Gain=-40
  Gain2 : Gain  Gain=10
  Gain3 : Gain  Gain=1-pressure_filter
  Gain4 : Gain  Gain=pressure_filter
  Gain5 : Gain  Gain=YAW_ENABLE
  Gain6 : Gain  Gain=[0.75 0.75 0.25 0.25]
  Gain7 : Gain  Gain=5
  Gain8 : Gain  Gain=[0.75 0.75 0.25 0.25]
  Product : Product
  Saturation : Saturate  UpperLimit=50  LowerLimit=0
  Saturation2 : Saturate  UpperLimit=Max_Brake_Pressure  LowerLimit=Min_Brake_Pressure
  Sum1 : Sum  Inputs=|++
  Sum2 : Sum  Inputs=|++
  Unit Delay1 : UnitDelay  SampleTime=-1  HasFrameUpgradeWarning=on
  Px : Outport
  wires:
  ABS_ENABLE/1 -> Product/1
  Saturation/1 -> Gain/1
  Sum1/1 -> Saturation/1
  Gain1/1 -> Sum1/1
  Gain2/1 -> Sum1/2
  <v_error>/1 -> Gain1/1
  omega/1 -> Discrete Derivative/1
  Discrete Derivative/1 -> Dead Zone/1
  Gain3/1 -> Sum2/2
  Gain/1 -> Gain6/1  "brake pressure"
  Unit Delay1/1 -> Gain3/1
  Gain4/1 -> Sum2/1
  Sum2/1 -> Product/2, Unit Delay1/1  "filtered brake pressure"
  Product/1 -> Saturation2/1
  Gain5/1 -> Gain4/1
  Gain6/1 -> Bias/1
  Dead Zone/1 -> Gain2/1
  In3/1 -> Abs/1
  Abs/1 -> 2-D Lookup Table/1
  In2/1 -> 2-D Lookup Table/2
  2-D Lookup Table/1 -> Gain7/1
  Saturation2/1 -> Px/1
  Gain7/1 -> Gain8/1
  Gain8/1 -> Gain5/1

== system car_model/Driver & Environment/Longitudinal Control/Pedal Positioner ==
  note: Determine when it is ok to trigger braking. If velocity error less than 0 (want to brake) and driver input is 0 (ready to brake) then it is ok to trigger brake
  <v_error> : Inport
  driver_input : Inport  Port=2
  AND : Logic  IconShape=distinctive  AllPortsSameDT=off  OutDataTypeStr=boolean
  Constant6 : Constant  Value=0
  Less Than1 : RelationalOperator  Operator=<=  OutDataTypeStr=boolean  RndMeth=Simplest  InputSameDT=off
  Less Than2 : RelationalOperator  Operator=<  OutDataTypeStr=boolean  RndMeth=Simplest  InputSameDT=off
  Unit Delay1 : UnitDelay  SampleTime=-1  HasFrameUpgradeWarning=on
  brake : Outport
  wires:
  Constant6/1 -> Less Than2/2, Less Than1/2
  AND/1 -> Unit Delay1/1
  Unit Delay1/1 -> brake/1
  Less Than2/1 -> AND/2
  <v_error>/1 -> Less Than2/1
  Less Than1/1 -> AND/1
  driver_input/1 -> Less Than1/1

== system car_model/Driver & Environment/Reference Generator/Subsystem ==
  <psi> : Inport
  Constant1 : Constant  Value=2*pi
  Constant2 : Constant  Value=pi
  Constant3 : Constant  Value=-pi
  Constant4 : Constant  Value=2*pi
  Constant5 : Constant  Value=-2*pi
  GreaterThan : RelationalOperator  Operator=>  OutDataTypeStr=boolean  RndMeth=Simplest  InputSameDT=off
  Less Than : RelationalOperator  Operator=<  OutDataTypeStr=boolean  RndMeth=Simplest  InputSameDT=off
  Mod : Math  Operator=mod
  Product : Product
  Product1 : Product
  Sum : Sum  Inputs=+++
  psi_rev : Outport
  wires:
  Product1/1 -> Sum/3
  Less Than/1 -> Product1/2
  GreaterThan/1 -> Product/1
  Mod/1 -> GreaterThan/1, Sum/1, Less Than/1
  Constant1/1 -> Mod/2
  Constant5/1 -> Product/2
  Constant3/1 -> Less Than/2
  Constant4/1 -> Product1/1
  Constant2/1 -> GreaterThan/2
  Product/1 -> Sum/2
  Sum/1 -> psi_rev/1
  <psi>/1 -> Mod/1
